simulink model "open_loop_test"  (Simulink 10.2)
settings: Solver=ode4  StartTime=0.0  StopTime=TMax  FixedStep=DT  MaxStep=DT  RelTol=1e-3  EnableMultiTasking=on
undefined symbols (not defined in the file or in its folder): OutList, strmatch
settings Model: Creator=bjonkman  LastModifiedBy=devin
settings DataIOCC: LimitDataPoints=on  SaveOutput=off  SaveTime=off  SignalLoggingName=sigsOut
settings OptimizationCC: ExpressionDepthLimit=2147483647
settings DebuggingCC: SaveWithParameterizedLinksMsg=none  SignalResolutionControl=TryResolveAllWithWarning  InheritedTsInSrcMsg=none  MultiTaskDSMMsg=warning  MultiTaskCondExecSysMsg=none  StateNameClashWarn=warning
settings HardwareCC: TargetUnknown=on

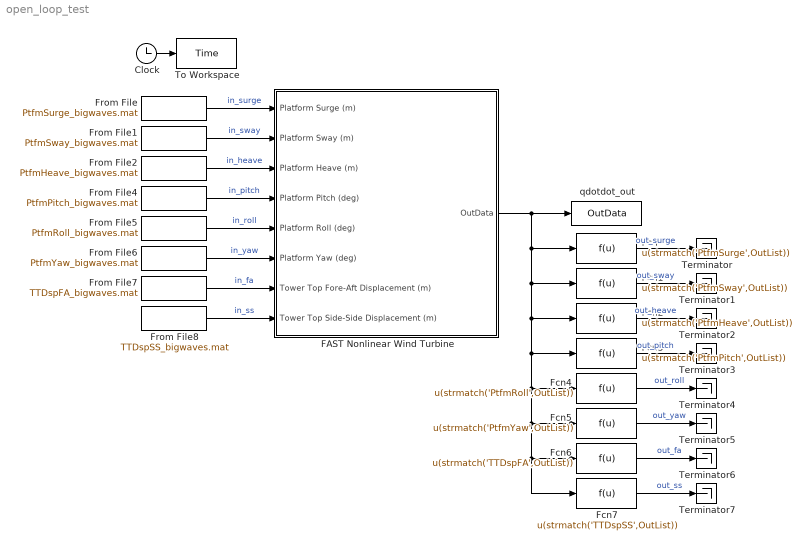
== system open_loop_test ==
  Clock : Clock
  FAST Nonlinear Wind Turbine : Subsystem  mask(FAST Nonlinear Wind Turbine){}
      mask help: This block contains the FAST S-Function.
      mask init:
      | clear FAST_SFunc
  Fcn : Fcn  Expr=u(strmatch('PtfmSurge',OutList))
  Fcn1 : Fcn  Expr=u(strmatch('PtfmSway',OutList))
  Fcn2 : Fcn  Expr=u(strmatch('PtfmHeave',OutList))
  Fcn3 : Fcn  Expr=u(strmatch('PtfmPitch',OutList))
  Fcn4 : Fcn  Expr=u(strmatch('PtfmRoll',OutList))
  Fcn5 : Fcn  Expr=u(strmatch('PtfmYaw',OutList))
  Fcn6 : Fcn  Expr=u(strmatch('TTDspFA',OutList))
  Fcn7 : Fcn  Expr=u(strmatch('TTDspSS',OutList))
  From File : FromFile  FileName=PtfmSurge_bigwaves.mat  SampleTime=.01
  From File1 : FromFile  FileName=PtfmSway_bigwaves.mat
  From File2 : FromFile  FileName=PtfmHeave_bigwaves.mat
  From File4 : FromFile  FileName=PtfmPitch_bigwaves.mat
  From File5 : FromFile  FileName=PtfmRoll_bigwaves.mat
  From File6 : FromFile  FileName=PtfmYaw_bigwaves.mat
  From File7 : FromFile  FileName=TTDspFA_bigwaves.mat
  From File8 : FromFile  FileName=TTDspSS_bigwaves.mat
  Terminator{,1..7} (8 alike) : Terminator
  To Workspace : ToWorkspace  VariableName=Time  SampleTime=-1
  qdotdot_out : ToWorkspace  VariableName=OutData  SampleTime=-1
  wires:
  Clock/1 -> To Workspace/1
  From File/1 -> FAST Nonlinear Wind Turbine/1(Platform Surge (m))  "in_surge"
  From File8/1 -> FAST Nonlinear Wind Turbine/8(Tower Top Side-Side Displacement (m))  "in_ss"
  From File7/1 -> FAST Nonlinear Wind Turbine/7(Tower Top Fore-Aft Displacement (m))  "in_fa"
  From File6/1 -> FAST Nonlinear Wind Turbine/6(Platform Yaw (deg))  "in_yaw"
  From File5/1 -> FAST Nonlinear Wind Turbine/5(Platform Roll (deg))  "in_roll"
  From File4/1 -> FAST Nonlinear Wind Turbine/4(Platform Pitch (deg))  "in_pitch"
  From File2/1 -> FAST Nonlinear Wind Turbine/3(Platform Heave (m))  "in_heave"
  From File1/1 -> FAST Nonlinear Wind Turbine/2(Platform Sway (m))  "in_sway"
  FAST Nonlinear Wind Turbine/1(OutData) -> Fcn7/1, Fcn6/1, Fcn5/1, Fcn4/1, Fcn3/1, Fcn2/1, Fcn1/1, Fcn/1, qdotdot_out/1
  Fcn/1 -> Terminator/1  "out_surge"
  Fcn7/1 -> Terminator7/1  "out_ss"
  Fcn1/1 -> Terminator1/1  "out_sway"
  Fcn6/1 -> Terminator6/1  "out_fa"
  Fcn5/1 -> Terminator5/1  "out_yaw"
  Fcn4/1 -> Terminator4/1  "out_roll"
  Fcn3/1 -> Terminator3/1  "out_pitch"
  Fcn2/1 -> Terminator2/1  "out_heave"

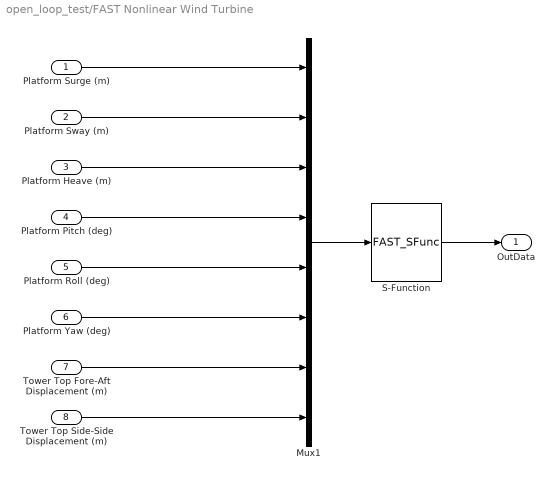
== system open_loop_test/FAST Nonlinear Wind Turbine ==
  Platform Surge (m) : Inport
  Platform Sway (m) : Inport  Port=2
  Platform Heave (m) : Inport  Port=3
  Platform Pitch (deg) : Inport  Port=4
  Platform Roll (deg) : Inport  Port=5
  Platform Yaw (deg) : Inport  Port=6
  Tower Top Fore-Aft Displacement (m) : Inport  Port=7
  Tower Top Side-Side Displacement (m) : Inport  Port=8
  Mux1 : Mux  Inputs=8
  S-Function : S-Function  FunctionName=FAST_SFunc  Parameters=FAST_InputFileName, TMax, 0  SFunctionDeploymentMode=off  EnableBusSupport=off
  OutData : Outport
  wires:
  S-Function/1 -> OutData/1
  Mux1/1 -> S-Function/1
  Platform Surge (m)/1 -> Mux1/1
  Platform Sway (m)/1 -> Mux1/2
  Platform Heave (m)/1 -> Mux1/3
  Platform Pitch (deg)/1 -> Mux1/4
  Platform Roll (deg)/1 -> Mux1/5
  Platform Yaw (deg)/1 -> Mux1/6
  Tower Top Fore-Aft Displacement (m)/1 -> Mux1/7
  Tower Top Side-Side Displacement (m)/1 -> Mux1/8
